simulink library "lwr_dynamics"  (Simulink 8.2)
settings: Solver=ode45  SolverMode=SingleTasking  StartTime=0.0  StopTime=10.0  RelTol=1e-3
libraries: lwr_dynamics x1
settings Model: Creator=krie_ka  LastModifiedBy=system  ExtModeAutoUpdateStatusClock=off

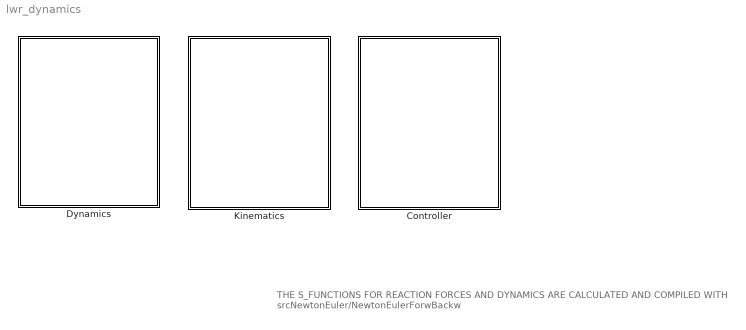
== system lwr_dynamics ==
  note: THE S_FUNCTIONS FOR REACTION FORCES AND DYNAMICS
      | ARE CALCULATED AND COMPILED WITH
      | srcNewtonEuler/NewtonEulerForwBackw
  Controller : Subsystem
      mask Display:
      | plot([0.3 0.3 0.7 0.7 0.3], [0.6 0.8 0.8 0.6 0.6]);
      | text(0.35, 0.71, 'xd = f(x,u)');
      | 
      | 
      | plot([0 0.2], [0.7 0.7]);
      | plot([0.3 0.2 0.2 0.3], [0.7 0.77 0.63 0.7]);
      | text(0.1, 0.82, 'u');
      | plot([0.7 0.9], [0.7 0.7]);
      | plot([1 0.9 0.9 1], [0.7 0.77 0.63 0.7]);
      | text(0.85, 0.82, 'x');
      | 
      | plot([0.3 0.3 0.7 0.7 0.3], [0.2 0.4 0.4 0.2 0.2]);
      | text(0.48, 0.32, 'K')
      | plot([0.7 0.75 0.75 0.7], [0.3 0.27 0.33 0.3]);
      | plot([0.75 0.8 0.8], [0.3 0.3 0.7])
      | plot([0.3 0.1 0.1], [0.3 0.3 0.65])
      | plot([0.1 0.07 0.13 0.1], [0.7 0.65 0.65 0.7]);
      | text(0.15, 0.6, '-');
  Dynamics : Subsystem
      mask Display:
      | plot([0.25 0.25 0.75 0.75 0.25], [0.25 0.75 0.75 0.25 0.25]);
      | text(0.35, 0.51, 'xd = f(x,u)');
      | 
      | plot([0 0.15], [0.5 0.5]);
      | plot([0.25 0.15 0.15 0.25], [0.5 0.57 0.43 0.5]);
      | text(0.1, 0.62, 'u');
      | plot([0.75 0.9], [0.5 0.5]);
      | plot([1 0.9 0.9 1], [0.5 0.57 0.43 0.5]);
      | text(0.85, 0.62, 'x');
  Kinematics : Subsystem
      mask Display:
      | plot(-0.15,-0.15);
      | plot(1.35,1.35);
      | plot([0 0.8 0.8 0.8 1 0.8],[0 0 0.1 -0.1 0 0.1]);
      | plot([0 0 0.1 -0.1 0 0.1],[0 0.8 0.8 0.8 1 0.8]);
      | text(1.15,0.05,'X');
      | text(0.02,1.15,'Z');
      | text(0.9,0.5,'Y');
      | plot([0, 0.6582, 0.7057, 0.6107, 0.8227, 0.7057],[0, 0.38, 0.2977, 0.4623, 0.475, 0.2977]);

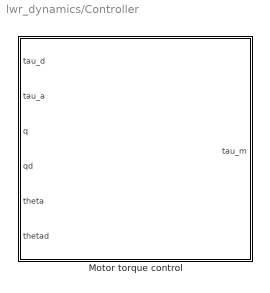
== system lwr_dynamics/Controller ==
  Motor torque control : Subsystem  mask{KJoint=[6900 10854.7 10000 10000 6464.3 10000 10000], DSJoint=20*ones(1,7), BJoint=[4.155 4.155 3.616 1.385 0.541 0.60083 0.60083], BThetaJoint=[4.155 4.155 3.616 1.385 0.541 0.60083 0.60083]/5}
      mask prompts: KJoint "Stiffness of joints"; DSJoint "Desired damping of Joints"; BJoint "Inertia of motorside"; BThetaJoint "Desired Inertia of motorside"
      mask Display:
      | image(imread('lbrjoint.jpg'))
      | port_label('input', 1, 'tau_des');
      | port_label('input', 2, 'tau_a');
      | port_label('input', 3, 'q');
      | port_label('input', 4, 'dq/dt');
      | port_label('input', 5, 'theta');
      | port_label('input', 6, 'dtheta/dt');
      | port_label('output', 1, 'tau_m');

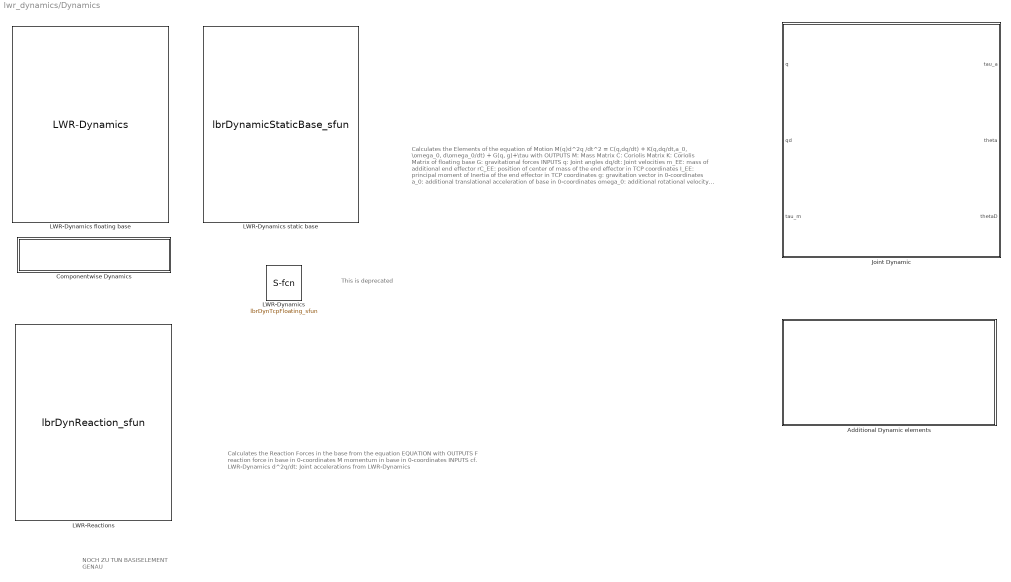
== system lwr_dynamics/Dynamics ==
  note: NOCH ZU TUN
      | BASISELEMENT GENAU
  note: Calculates the Elements of the equation of Motion
      | M(q)d^2q /dt^2 = C(q,dq/dt) + K(q,dq/dt,a_0, \omega_0, d\omega_0/dt) + G(q, g)+\tau
      | with
      | OUTPUTS
      |    M: Mass Matrix
      |    C: Coriolis Matrix
      |    K: Coriolis Matrix of floating base
      |    G: gravitational forces
      | INPUTS
      |    q: Joint angles
      |    dq/dt: Joint velocities
      |    m_EE: mass of additional end effector
      |    rC_EE: position of center of mass of the end effector in TCP coordinates
      |    I_EE:  principal moment of Inertia of the end effector in TCP coordinates
      |    g: gravitation vector in 0-coordinates
      |    a_0: additional translational acceleration of base in 0-coordinates
      |    omega_0: additional rotational velocity of base in 0-coordinates
      |    domega_0/dt additional rotational acceleration of base in 0-coordnates
  note: Calculates the Reaction Forces in the base from the equation
      | EQUATION
      | with
      | OUTPUTS
      |     F reaction force in base in 0-coordinates
      |     M momentum in base in 0-coordinates
      | INPUTS
      |    cf. LWR-Dynamics
      |    d^2q/dt: Joint accelerations from LWR-Dynamics
  note: This is deprecated
  Additional Dynamic elements : Subsystem
  Componentwise Dynamics : Subsystem
  Joint Dynamic : Subsystem
      mask Display:
      | image(imread('lbrjoint.jpg'))
      | port_label('input', 1, 'q')
      | port_label('input', 2, 'dq/dt')
      | port_label('input', 3, 'tau_m')
      | port_label('output', 1, 'tau_a')
      | port_label('output', 2, 'theta')
      | port_label('output', 3, 'dtheta/dt')
      | port_label('output', 4, 'tau')
  LWR-Dynamics : S-Function  FunctionName=lbrDynTcpFloating_sfun  EnableBusSupport=off
      mask Display:
      | image(imread('lbr.jpg'));
      | port_label('input', 1, 'q');
      | port_label('input', 2, 'dq/dt');
      | port_label('input', 3, 'm_EE');
      | port_label('input', 4, 'rC_EE');
      | port_label('input', 5, 'I_EE');
      | port_label('input', 6, 'g');
      | port_label('input', 7, 'a_0');
      | port_label('input', 8, 'omega_0');
      | port_label('input', 9, 'domega_0/dt');
      | 
      | port_label('output', 1, 'G');
      | port_label('output', 2, 'C');
      | port_label('output', 3, 'K');
      | port_label('output', 4, 'M');
  LWR-Dynamics floating base : lwr_dynamics/Dynamics/LWR-Dynamics
  LWR-Dynamics static base : S-Function  FunctionName=lbrDynamicStaticBase_sfun  EnableBusSupport=off
      mask Display:
      | image(imread('lbr.jpg'));
      | port_label('input', 1, 'q');
      | port_label('input', 2, 'dq/dt');
      | port_label('input', 3, 'm_EE');
      | port_label('input', 4, 'rC_EE');
      | port_label('input', 5, 'I_EE');
      | port_label('input', 6, 'g');
      | 
      | 
      | port_label('output', 1, 'G');
      | port_label('output', 2, 'C');
      | port_label('output', 3, 'M');
  LWR-Reactions : S-Function  FunctionName=lbrDynReaction_sfun  EnableBusSupport=off
      mask Display:
      | image(imread('lbr.jpg'));
      | port_label('input', 1, 'q');
      | port_label('input', 2, 'dq/dt');
      | port_label('input', 3, 'd^2q/dt^2');
      | port_label('input', 4, 'm_EE');
      | port_label('input', 5, 'rC_EE');
      | port_label('input', 6, 'I_EE');
      | port_label('input', 7, 'g');
      | port_label('input', 8, 'a_0');
      | port_label('input', 9, 'omega_0');
      | port_label('input', 10, 'domega_0/dt');
      | 
      | port_label('output', 1, 'F');
      | port_label('output', 2, 'M');

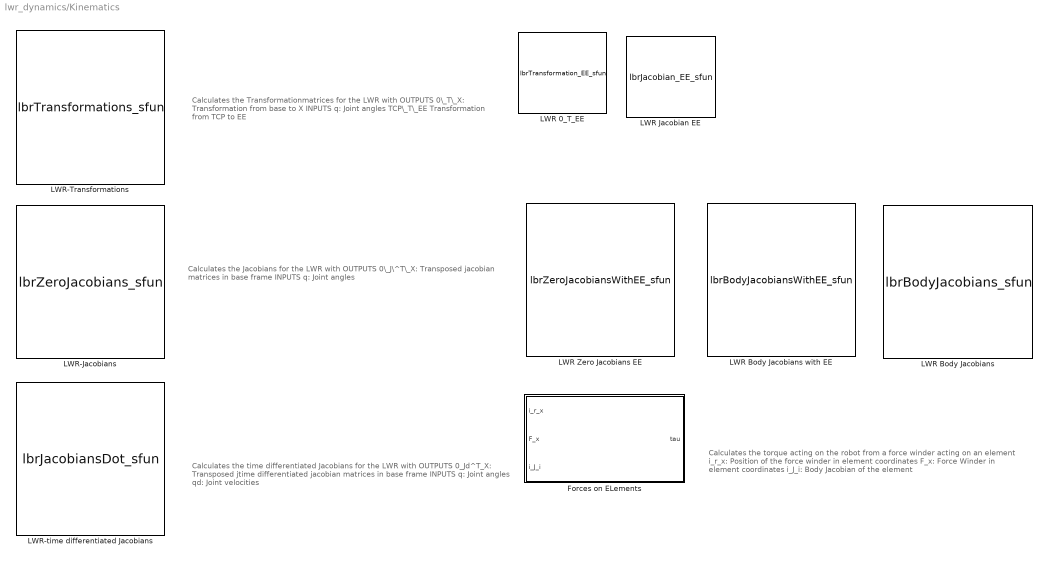
== system lwr_dynamics/Kinematics ==
  note: Calculates the Transformationmatrices for the LWR
      |
      | with
      | OUTPUTS
      |    0\_T\_X: Transformation from base to X
      | INPUTS
      |    q: Joint angles
      |    TCP\_T\_EE Transformation from TCP to EE
  note: Calculates the Jacobians for the LWR
      |
      | with
      | OUTPUTS
      |    0\_J\^T\_X: Transposed jacobian matrices in base frame
      | INPUTS
      |    q: Joint angles
  note: Calculates the time differentiated Jacobians for the LWR
      |
      | with
      | OUTPUTS
      |    0_Jd^T_X: Transposed jtime differentiated
      |                      jacobian matrices in base frame
      | INPUTS
      |    q: Joint angles
      |    qd: Joint velocities
  note: Calculates the torque acting on the robot  from a
      | force winder acting on an element
      |
      | i_r_x: Position of the force winder in element coordinates
      | F_x: Force Winder in element coordinates
      | i_J_i: Body Jacobian of the element
  Forces on ELements : MATLAB Function  TreatAsAtomicUnit=on
  LWR 0_T_EE : S-Function  FunctionName=lbrTransformation_EE_sfun  EnableBusSupport=off
      mask Display:
      | image(imread('lbr.jpg'));
      | port_label('input', 1, 'q');
      | port_label('input', 2, '7_T_EE');
      | 
      | 
      | port_label('output', 1, '0_T_EE');
  LWR Body Jacobians : S-Function  FunctionName=lbrBodyJacobians_sfun  EnableBusSupport=off
      mask Display:
      | image(imread('lbr.jpg'));
      | port_label('input', 1, 'q');
      | 
      | 
      | 
      | port_label('output', 1, '1_J^T_1');
      | port_label('output', 2, '2_J^T_2');
      | port_label('output', 3, '3_J^T_3');
      | port_label('output', 4, '4_J^T_4');
      | port_label('output', 5, '5_J^T_5');
      | port_label('output', 6, '6_J^T_6');
      | port_label('output', 7, '7_J^T_7');
  LWR Body Jacobians with EE : S-Function  FunctionName=lbrBodyJacobiansWithEE_sfun  EnableBusSupport=off
      mask Display:
      | image(imread('lbr.jpg'));
      | port_label('input', 1, 'q');
      | port_label('input', 2, '7_T_EE');
      | 
      | 
      | port_label('output', 1, '1_J^T_1');
      | port_label('output', 2, '2_J^T_2');
      | port_label('output', 3, '3_J^T_3');
      | port_label('output', 4, '4_J^T_4');
      | port_label('output', 5, '5_J^T_5');
      | port_label('output', 6, '6_J^T_6');
      | port_label('output', 7, '7_J^T_7');
      | port_label('output', 8, 'EE_J^T_EE');
  LWR Jacobian EE : S-Function  FunctionName=lbrJacobian_EE_sfun  EnableBusSupport=off
      mask Display:
      | image(imread('lbr.jpg'));
      | port_label('input', 1, 'q');
      | port_label('input', 2, '7_T_EE');
      | 
      | 
      | port_label('output', 1, '0_J^T_EE');
  LWR Zero Jacobians EE : S-Function  FunctionName=lbrZeroJacobiansWithEE_sfun  EnableBusSupport=off
      mask Display:
      | image(imread('lbr.jpg'));
      | port_label('input', 1, 'q');
      | port_label('input', 2, '7_T_EE');
      | 
      | port_label('output', 1, '0_J^T_1');
      | port_label('output', 2, '0_J^T_2');
      | port_label('output', 3, '0_J^T_3');
      | port_label('output', 4, '0_J^T_4');
      | port_label('output', 5, '0_J^T_5');
      | port_label('output', 6, '0_J^T_6');
      | port_label('output', 7, '0_J^T_7');
      | port_label('output', 8, '0_J^T_EE');
  LWR-Jacobians : S-Function  FunctionName=lbrZeroJacobians_sfun  EnableBusSupport=off
      mask Display:
      | image(imread('lbr.jpg'));
      | port_label('input', 1, 'q');
      | 
      | 
      | 
      | port_label('output', 1, '0_J^T_1');
      | port_label('output', 2, '0_J^T_2');
      | port_label('output', 3, '0_J^T_3');
      | port_label('output', 4, '0_J^T_4');
      | port_label('output', 5, '0_J^T_5');
      | port_label('output', 6, '0_J^T_6');
      | port_label('output', 7, '0_J^T_7');
  LWR-Transformations : S-Function  FunctionName=lbrTransformations_sfun  EnableBusSupport=off
      mask Display:
      | image(imread('lbr.jpg'));
      | port_label('input', 1, 'q');
      | port_label('input', 2, '7_T_EE');
      | 
      | 
      | port_label('output', 1, '0_T_1');
      | port_label('output', 2, '0_T_2');
      | port_label('output', 3, '0_T_3');
      | port_label('output', 4, '0_T_4');
      | port_label('output', 5, '0_T_5');
      | port_label('output', 6, '0_T_6');
      | port_label('output', 7, '0_T_7');
      | port_label('output', 8, '0_T_EE');
  LWR-time differentiated Jacobians : S-Function  FunctionName=lbrJacobiansDot_sfun  EnableBusSupport=off
      mask Display:
      | image(imread('lbr.jpg'));
      | port_label('input', 1, 'q');
      | port_label('input', 2, 'qd');
      | 
      | 
      | port_label('output', 1, '0_Jd^T_1');
      | port_label('output', 2, '0_Jd^T_2');
      | port_label('output', 3, '0_Jd^T_3');
      | port_label('output', 4, '0_Jd^T_4');
      | port_label('output', 5, '0_Jd^T_5');
      | port_label('output', 6, '0_Jd^T_6');
      | port_label('output', 7, '0_Jd^T_7');

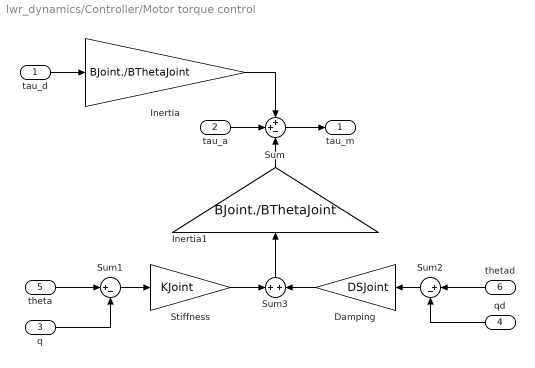
== system lwr_dynamics/Controller/Motor torque control ==
  tau_d : Inport
  tau_a : Inport  Port=2
  q : Inport  Port=3
  qd : Inport  Port=4
  theta : Inport  Port=5
  thetad : Inport  Port=6
  Damping : Gain  Gain=DSJoint
  Inertia : Gain  Gain=BJoint./BThetaJoint
  Inertia1 : Gain  Gain=BJoint./BThetaJoint
  Stiffness : Gain  Gain=KJoint
  Sum : Sum  Inputs=++-
  Sum1 : Sum  Inputs=|+-
  Sum2 : Sum  Inputs=|+-
  Sum3 : Sum
  tau_m : Outport
  wires:
  tau_d/1 -> Inertia/1
  Sum/1 -> tau_m/1
  tau_a/1 -> Sum/2
  Inertia/1 -> Sum/1
  Inertia1/1 -> Sum/3
  theta/1 -> Sum1/1
  q/1 -> Sum1/2
  thetad/1 -> Sum2/1
  qd/1 -> Sum2/2
  Sum3/1 -> Inertia1/1
  Sum1/1 -> Stiffness/1
  Sum2/1 -> Damping/1
  Stiffness/1 -> Sum3/1
  Damping/1 -> Sum3/2

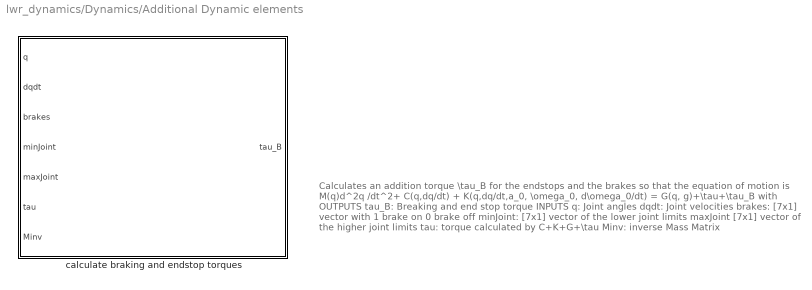
== system lwr_dynamics/Dynamics/Additional Dynamic elements ==
  note: Calculates an addition torque \tau_B for the endstops and the brakes so that the equation of motion is
      | M(q)d^2q /dt^2+ C(q,dq/dt) + K(q,dq/dt,a_0, \omega_0, d\omega_0/dt) = G(q, g)+\tau+\tau_B
      | with
      | OUTPUTS
      |    tau_B: Breaking and end stop torque
      | INPUTS
      |    q: Joint angles
      |    dqdt: Joint velocities
      |    brakes: [7x1] vector with 1 brake on 0 brake off
      |    minJoint: [7x1] vector of the lower joint limits
      |    maxJoint [7x1] vector  of the higher joint limits
      |    tau: torque calculated by C+K+G+\tau
      |    Minv: inverse Mass Matrix
  calculate braking and endstop torques : MATLAB Function  TreatAsAtomicUnit=on

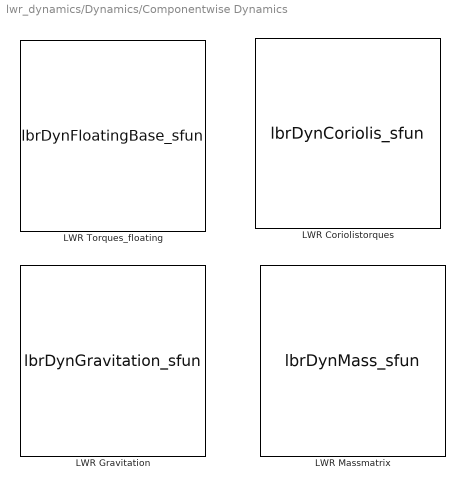
== system lwr_dynamics/Dynamics/Componentwise Dynamics ==
  LWR Coriolistorques : S-Function  FunctionName=lbrDynCoriolis_sfun  EnableBusSupport=off
      mask Display:
      | image(imread('lbr.jpg'));
      | port_label('input', 1, 'q');
      | port_label('input', 2, 'qd');
      | port_label('input', 3, 'm_EE');
      | port_label('input', 4, 'r_EE');
      | port_label('input', 5, 'I_EE');
      | 
      | 
      | port_label('output', 1, 'tau_coriolis');
  LWR Gravitation : S-Function  FunctionName=lbrDynGravitation_sfun  EnableBusSupport=off
      mask Display:
      | image(imread('lbr.jpg'));
      | port_label('input', 1, 'q');
      | port_label('input', 2, 'm_EE');
      | port_label('input', 3, 'r_EE');
      | port_label('input', 4, 'g');
      | 
      | port_label('output', 1, 'tau_gravity');
  LWR Massmatrix : S-Function  FunctionName=lbrDynMass_sfun  EnableBusSupport=off
      mask Display:
      | image(imread('lbr.jpg'));
      | port_label('input', 1, 'q');
      | port_label('input', 2, 'm_EE');
      | port_label('input', 3, 'r_EE');
      | port_label('input', 4, 'I_EE');
      | 
      | port_label('output', 1, 'M');
  LWR Torques_floating : S-Function  FunctionName=lbrDynFloatingBase_sfun  EnableBusSupport=off
      mask Display:
      | image(imread('lbr.jpg'));
      | port_label('input', 1, 'q');
      | port_label('input', 2, 'qd');
      | port_label('input', 3, 'm_EE');
      | port_label('input', 4, 'r_EE');
      | port_label('input', 5, 'I_EE');
      | port_label('input', 6, 'a_0');
      | port_label('input', 7, 'omega_0');
      | port_label('input', 8, 'domega_0/dt');
      | 
      | port_label('output', 1, 'tau_floating');

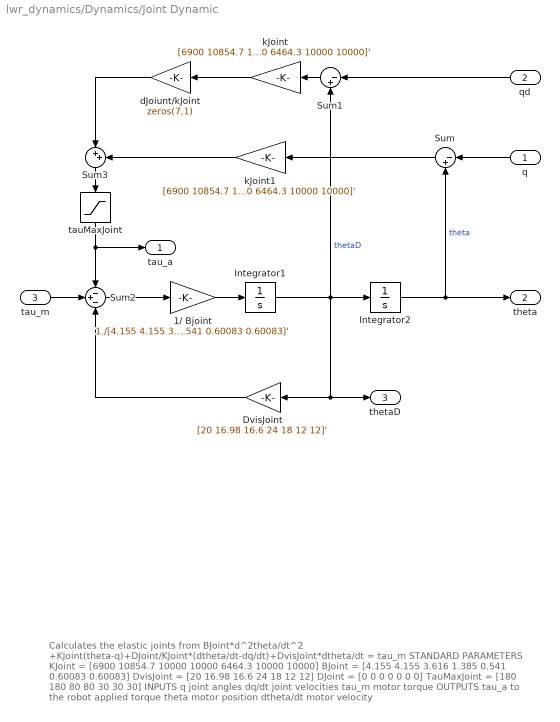
== system lwr_dynamics/Dynamics/Joint Dynamic ==
  note: Calculates the elastic joints from
      | BJoint*d^2theta/dt^2 +KJoint(theta-q)+DJoint/KJoint*(dtheta/dt-dq/dt)+DvisJoint*dtheta/dt = tau_m
      |
      | STANDARD PARAMETERS
      | KJoint = [6900 10854.7 10000 10000 6464.3 10000 10000]
      | BJoint = [4.155 4.155 3.616 1.385 0.541 0.60083 0.60083]
      | DvisJoint = [20 16.98 16.6 24 18 12 12]
      | DJoint = [0 0 0 0 0 0 0]
      | TauMaxJoint = [180 180 80 80 30 30 30]
      |
      | INPUTS
      |    q joint angles
      |    dq/dt joint velocities
      |    tau_m motor torque
      |
      | OUTPUTS
      |    tau_a to the robot applied torque
      |    theta motor position
      |    dtheta/dt motor velocity
  q : Inport
  qd : Inport  Port=2
  tau_m : Inport  Port=3
  1/ Bjoint : Gain  Gain=1./[4.155 4.155 3.616 1.385 0.541 0.60083 0.60083]'
  DvisJoint : Gain  Gain=[20 16.98 16.6 24 18 12 12]'
  Integrator1 : Integrator  InitialCondition=zeros(7,1)
  Integrator2 : Integrator  InitialCondition=zeros(7,1)
  Sum : Sum  Inputs=|-+
  Sum1 : Sum  Inputs=|-+
  Sum2 : Sum  Inputs=-+-
  Sum3 : Sum  Inputs=|++
  dJoiunt/kJoint : Gain  Gain=zeros(7,1)
  kJoint : Gain  Gain=[6900 10854.7 10000 10000 6464.3 10000 10000]'
  kJoint1 : Gain  Gain=[6900 10854.7 10000 10000 6464.3 10000 10000]'
  tauMaxJoint : Saturate  UpperLimit=[180 180 80 80 30 30 30]'  LowerLimit=-[180 180 80 80 30 30 30]'
  tau_a : Outport
  theta : Outport  Port=2
  thetaD : Outport  Port=3
  wires:
  Integrator1/1 -> Sum1/2, Integrator2/1, DvisJoint/1, thetaD/1  "thetaD"
  q/1 -> Sum/1
  Integrator2/1 -> Sum/2, theta/1  "theta"
  qd/1 -> Sum1/1
  Sum2/1 -> 1/ Bjoint/1
  tau_m/1 -> Sum2/2
  Sum/1 -> kJoint1/1
  Sum1/1 -> kJoint/1
  kJoint1/1 -> Sum3/2
  dJoiunt/kJoint/1 -> Sum3/1
  DvisJoint/1 -> Sum2/3
  1/ Bjoint/1 -> Integrator1/1
  Sum3/1 -> tauMaxJoint/1
  tauMaxJoint/1 -> Sum2/1, tau_a/1
  kJoint/1 -> dJoiunt/kJoint/1

== matlab function Kinematics/Forces on ELements ==
  data: i_r_x input double size=3; tau output double size=7; F_x input double size=6; i_J_i input double size=[7 6]
function tau = calcTorque(i_r_x, F_x, i_J_i)


tau = i_J_i* [eye(3,3)                     zeros(3,3)
              [0       -i_r_x(3) i_r_x(2)
               i_r_x(3) 0       -i_r_x(1)
              -i_r_x(2) i_r_x(1) 0       ] eye(3,3)] * F_x;

== matlab function Dynamics/Additional Dynamic elements/calculate braking and endstop torques ==
  data: q input double size=7; dqdt input double size=7; brakes input double size=7; minJoint input double size=7; maxJoint input double size=7; tau_B output double size=7; tau input double size=7; Minv input double size=[7 7]
function tau_B = calcBrakesAndEndStops(q, dqdt, brakes, minJoint, maxJoint, tau, Minv)
    
    I = eye(7,7);
    brakedamping=2*ones(7,1);
    null = zeros(7,1);
    j = 0;  % Nr of active Breaks
    chooseR = zeros(7,7);  % Choose Matrix
    qEnd = zeros(7,1);
    activeEndStops = zeros(7,1);
    MinvTau = Minv*tau;
    pole1 = 40;
    pole2 = 40;
    
    
    % CALCULATE ENDSTOP TORQUES
    %#######################################
    for i=1:7
        if (q(i) > maxJoint(i) && brakes(i) ~= 1)
            tau_test = Minv*brake(I(i,:), I(:,i), dqdt, tau, Minv, pole1*pole2*I(:,i), (pole1+pole2)*I(:,i), q, I(:,i)*maxJoint(i));
            if (MinvTau(i) > tau_test(i)) 
                qEnd(i) = maxJoint(i);
                activeEndStops(i) = 1;
                j = j+1;
                chooseR(j,:) = I(i,:);
            end
        end
        if (q(i) < minJoint(i) && brakes(i) ~= 1)
           tau_test = Minv*brake(I(i,:), I(:,i), dqdt, tau, Minv, pole1*pole2*I(:,i), (pole1+pole2)*I(:,i), q, I(:,i)*maxJoint(i));
           if (MinvTau(i) < tau_test(i)) 
                qEnd(i) = minJoint(i);
                activeEndStops(i) = 1;
                j = j+1;
                chooseR(j,:) = I(i,:);
           end
        end
    end  

    
    K = activeEndStops*pole1*pole2;
    D = activeEndStops*(pole1+pole2);
    
    % How much Joints are in End Stop
    switch j
        case 1
            tau_end = brake(chooseR(1,:),   activeEndStops, dqdt, tau, Minv, K, D, q, qEnd);
        case 2
            tau_end = brake(chooseR(1:2,:), activeEndStops, dqdt, tau, Minv, K, D, q, qEnd);
        case 3
            tau_end = brake(chooseR(1:3,:), activeEndStops, dqdt, tau, Minv, K, D, q, qEnd);
        case 4
            tau_end = brake(chooseR(1:4,:), activeEndStops, dqdt, tau, Minv, K, D, q, qEnd);
        case 5
            tau_end = brake(chooseR(1:5,:), activeEndStops, dqdt, tau, Minv, K, D, q, qEnd);
        case 6
            tau_end = brake(chooseR(1:6,:), activeEndStops, dqdt, tau, Minv, K, D, q, qEnd);
        case 7
            tau_end = brake(chooseR(1:7,:), activeEndStops, dqdt, tau, Minv, K, D, q, qEnd);
        otherwise   
           tau_end = zeros(7,1);
    end
    
    tau_B = tau_end;
    
    
    % CALCULATE BRAKING TORQUES
    %#######################################
    chooseR = zeros(7,7);
    j = 0;
    % Construct choosematrix
    for i=1:7
        if brakes(i) == 1
            j = j+1;
            chooseR(j,:) = I(i,:);
        end
    end
    tau = tau+tau_B; %reaction forces of end stops should not interfere the brakes
    
        
    % How much Joints are braked
    switch j
        case 1
            tau_brake = brake(chooseR(1,:),   brakes, dqdt, tau, Minv, null, brakedamping, null, null);
        case 2
            tau_brake = brake(chooseR(1:2,:), brakes, dqdt, tau, Minv, null, brakedamping, null, null);
        case 3
            tau_brake = brake(chooseR(1:3,:), brakes, dqdt, tau, Minv, null, brakedamping, null, null);
        case 4
            tau_brake = brake(chooseR(1:4,:), brakes, dqdt, tau, Minv, null, brakedamping, null, null);
        case 5
            tau_brake = brake(chooseR(1:5,:), brakes, dqdt, tau, Minv, null, brakedamping, null, null);
        case 6
            tau_brake = brake(chooseR(1:6,:), brakes, dqdt, tau, Minv, null, brakedamping, null, null);
        case 7
            tau_brake = brake(chooseR(1:7,:), brakes, dqdt, tau, Minv, null, brakedamping, null, null);
        otherwise   
           tau_brake = zeros(7,1);
    end
    
    tau_B = tau_B+tau_brake;
end

function tau = brake(choose, brakes, dqdt, tau, Minv, K, D, q, qdes)
     %Phi _q denotes the derivative of the reaction forces matrix and is [7xr] matrix (r denotes the number of braked joints)
    phi_q = choose*diag(brakes);
    
    multiplier = inv(phi_q*Minv*phi_q.');
    baumgarteStabilisierung = choose*(D.*dqdt)+choose*(K.*(q-qdes));
    tau = choose.'*(multiplier*(phi_q*Minv*(-tau))-baumgarteStabilisierung);
end
